simulink model "phase_modulator_simulation"  (R2017a)
settings: Solver=VariableStepAuto  StartTime=0.0  StopTime=.001  RelTol=1e-3
settings Model: Creator=Kilian  LastModifiedBy=Kilian

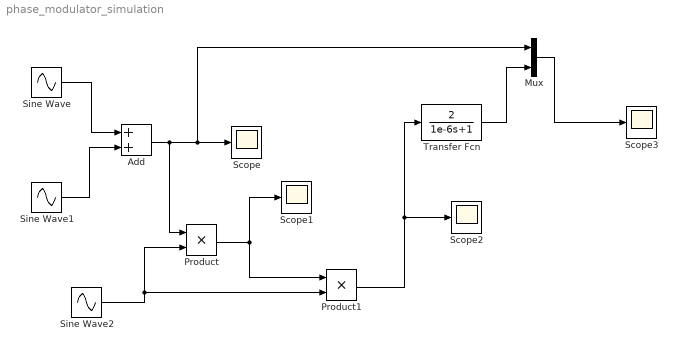
== system phase_modulator_simulation ==
  Add : Sum
  Mux : Mux  Inputs=2
  Product : Product
  Product1 : Product
  Scope{,1..3} (4 alike) : Scope
  Sine Wave : Sin  Frequency=2*pi*20000  SampleTime=0
  Sine Wave1 : Sin  Frequency=2*pi*21000  SampleTime=0
  Sine Wave2 : Sin  Frequency=2*pi*1.356*1e6  SampleTime=0
  Transfer Fcn : TransferFcn  Numerator=[2]  Denominator=[1e-6 1]
  wires:
  Sine Wave1/1 -> Add/2
  Sine Wave/1 -> Add/1
  Add/1 -> Mux/1, Scope/1, Product/1
  Sine Wave2/1 -> Product1/2, Product/2
  Product/1 -> Product1/1, Scope1/1
  Product1/1 -> Transfer Fcn/1, Scope2/1
  Transfer Fcn/1 -> Mux/2
  Mux/1 -> Scope3/1
